simulink model "prob5"  (R2020b)
settings: Solver=VariableStepAuto  StartTime=0.0  StopTime=10.0  RelTol=1e-3
values from neighbouring files (symbols this model uses):
  C = 0.01    [values.mat]
  R = 10    [values.mat]
settings Model: Creator=DELL  LastModifiedBy=DELL

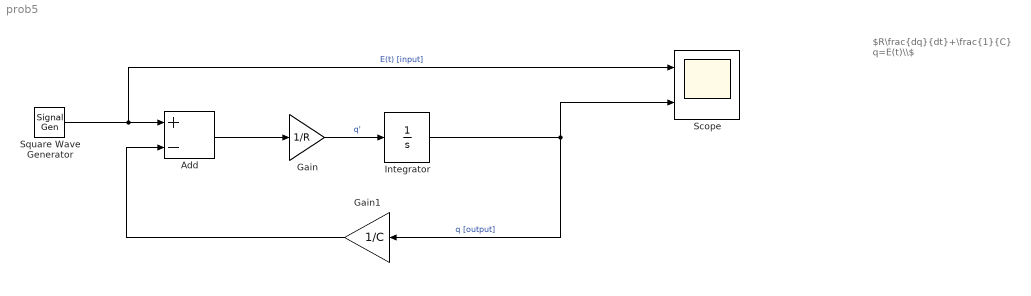
== system prob5 ==
  note: $R\frac{dq}{dt}+\frac{1}{C} q=E(t)\\$
  Add : Sum  Inputs=+-
  Gain : Gain  Gain=1/R
  Gain1 : Gain  Gain=1/C
  Integrator : Integrator
  Scope : Scope  NumInputPorts=2
  Square Wave Generator : SignalGenerator  WaveForm=square  Units=rad/sec
  wires:
  Add/1 -> Gain/1
  Gain/1 -> Integrator/1  "q'"
  Integrator/1 -> Scope/2, Gain1/1  "q [output]"
  Gain1/1 -> Add/2
  Square Wave Generator/1 -> Scope/1, Add/1  "E(t) [input]"
